simulink library "wcdma_lib"  (Simulink 6.0)
settings: Solver=ode45  SolverMode=SingleTasking  StartTime=0.0  StopTime=10.0  RelTol=1e-3
values from neighbouring files (symbols this model uses):
  allocationssc = [1 1 1 1 1 1 1 1 1 1 1 1 ... (960 elements, 64x15)]    [wcdma_allocationssc.mat]
  crcSize = str2num(Vals{idxCrcSize})    [wcdma_initmaskphlayer.m]    (also in wcdma_loadinitmuxandcoding.m = [16 12]; wcdma_loadinitphlayer.m = [16 12])
  errorCorr = (errorCorr>2)*2 + (errorCorr<3).*errorCorr    [wcdma_initmaskphlayer.m]    (also in wcdma_loadinitmuxandcoding.m = [2 2]; wcdma_loadinitphlayer.m = [2 2])
  i = [1:2:numSamp-1]'    [cdma2000_inttable.m]
  numBitsCodeWord = cond.*Zmin + not(cond).*numBitsCodeWord    [wcdma_concseg.m]    (also in wcdma_loadinitmuxandcoding.m = [260 122])
  numBitsFirstInt = numBitsRM + deltaNimax    [wcdma_initmaskphlayer.m]    (also in wcdma_loadinitmuxandcoding.m = [686 308])
  numBitsRF = numBitsFirstInt./(tti/10)    [wcdma_initmaskphlayer.m]    (also in wcdma_loadinitmuxandcoding.m = [343 77]; wcdma_loadinitphlayer.m = [343 77])
  numBitsTrCh = (trBlkSize+crcSize)*diag(numTrBlks)    [wcdma_concseg.m]    (also in wcdma_loadinitmuxandcoding.m = [260 112])
  numCodeWords = ceil(numBitsTrCh./Zmax(errorCorr+1))    [wcdma_concseg.m]    (also in wcdma_loadinitmuxandcoding.m = [1 1])
  numPadBits = (numBitsCodeWord.*numCodeWords)-numBitsTrCh    [wcdma_concseg.m]    (also in wcdma_loadinitmuxandcoding.m = [0 0])
  numPhCH = str2num(Vals{idxNumPhCH})    [wcdma_initmaskphlayer.m]    (also in wcdma_loadinitmuxandcoding.m = 1; wcdma_loadinitphlayer.m = 1)
  numTrBlks = trBlkSetSize./trBlkSize    [wcdma_concseg.m]    (also in wcdma_initmaskphlayer.m; wcdma_loadinitmuxandcoding.m = [1 1]; wcdma_loadinitphlayer.m = [1 1])
  overSampling = str2num(Vals{idxOverSampling})    [wcdma_initmaskphlayer.m]    (also in wcdma_initmaskspreadandmod.m; wcdma_loadinitphlayer.m = 8; wcdma_loadinitspreadandmod.m = 8)
  powerVector = str2num(Vals{idxPowerVector})    [wcdma_initmaskphlayer.m]    (also in wcdma_initmaskspreadandmod.m; wcdma_loadinitphlayer.m = [-5.5 -10 -15 -12 -12]; wcdma_loadinitspreadandmod.m = [-5.5 -10 -15 -12 -12])
  sprdFactor = wcdma_slotformattable(slotFormat+1,2)    [wcdma_checkparamstxant.m]    (also in wcdma_initmaskphlayer.m = slotformattable(slotFormat+1,2); wcdma_initmaskspreadandmod.m = slotformattable(slotFormat+1,2); wcdma_loadinitphlayer.m = 128; wcdma_loadinitspreadandmod.m = 128)
  tti = str2num(Vals{idxTti})    [wcdma_initmaskphlayer.m]    (also in wcdma_loadinitmuxandcoding.m = [20 40]; wcdma_loadinitphlayer.m = [20 40])
undefined symbols (not defined in the file or in its folder): hadamard, numSymbOut
libraries: wcdma_lib x122, dspsrcs4 x39, dspsigops x30, commseqgen2 x24, dspindex x20, dspbuff3 x19, dspmathops x16, simulink x10, dspsigattribs x7, commutil2 x6, dspmtrx3 x6, commblkintrlv2 x6
(part 1 of 3)
settings Model: Creator=arodrigu  LastModifiedBy=arodrigu  ProdHWDeviceType=Specified
settings DataIOCC: SignalLoggingName=logsOut
settings OptimizationCC: BooleanDataType=off
settings DebuggingCC: CheckExecutionContextPreStartOutputMsg=on  CheckExecutionContextRuntimeOutputMsg=on  SolverPrmCheckMsg=none
settings HardwareCC: ProdHWDeviceType=Specified  TargetUnknown=on
settings ModelReferenceCC: UpdateModelReferenceTargets=IfOutOfDate
settings GRTTargetCC: LifeSpan=inf
settings SFSimCC: SFSimApplyToAllLibs=on  SFSimBuildMode=Incremental

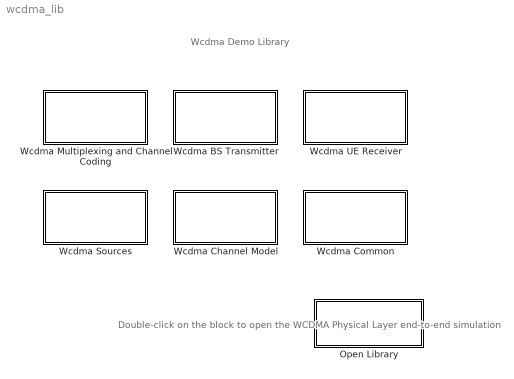
== system wcdma_lib ==
  note: Wcdma Demo Library
  note: Double-click on the block
      | to open the WCDMA Physical
      | Layer end-to-end simulation
  Open Library : Subsystem  EnableExecutionContextPropagation=on
      settings: OpenFcn=open('wcdma_phlayer.mdl');
      mask Display: disp('WCDMA PhLayer\nEnd-to-End\nSimulation')
  Wcdma BS Transmitter : Subsystem  EnableExecutionContextPropagation=on
      mask Type: Wcdma BS Tx
      mask Display: disp('Wcdma \nBS \nTransmitter');
  Wcdma Channel Model : Subsystem  EnableExecutionContextPropagation=on
      mask Type: Wcdma Common
      mask Display: disp('Wcdma \nChannel Model');
  Wcdma Common : Subsystem  EnableExecutionContextPropagation=on
      mask Type: Wcdma Common
      mask Display: disp('Wcdma \nCommon Blocks');
  Wcdma Multiplexing and Channel Coding : Subsystem  EnableExecutionContextPropagation=on
      mask Display: disp('Wcdma\nMultiplexing\nand Channel coding');
  Wcdma Sources : Subsystem  EnableExecutionContextPropagation=on
      mask Type: Wcdma Sources
      mask Display: disp('Wcdma \nSources');
  Wcdma UE Receiver : Subsystem  EnableExecutionContextPropagation=on
      mask Type: Wcdma UE Rx
      mask Display: disp('Wcdma \nUE \nReceiver');

== system wcdma_lib/Open Library ==
  note: This subsystem is intentionally left empty

== system wcdma_lib/Wcdma BS Transmitter ==
  note: Wcdma BS Transmitter
  Complex Spreading Multiplication : Subsystem  EnableExecutionContextPropagation=on  mask(Complex Spreading){sprdFactor=256}
      mask prompts: sprdFactor "Spreading Factor (SF):"
  Wcdma BS Tx Antenna : Subsystem  EnableExecutionContextPropagation=on  mask(Wcdma BS Tx Antenna){slotFormat=11, dpchCode=123, scrCode=[63 0], powerVector=[-8.8 -10 -15 -12 -12], numTapsRRC=96, overSampling=8, checkparams=off}
      mask prompts: slotFormat "Slot Format (0..16):"; dpchCode "DPCH Code number (0..Spreading Factor -1):"; scrCode "Scrambling Code [Scr Code Grup(0..63) Primary Code(0..7)]:"; powerVector "Power for [DPCH, P-CPICH, PICH, P-CCPCH, SCH] in dB:"; numTapsRRC "Number of Filter Taps for RRC filters:"; overSampling "Oversampling Factor:"; checkparams "Check here to validate parameters."
      mask help:
      | After combining the different transport channels into physical channels, data is sent to the Downlink Base Station Tranmitter Antenna in the form of slots.
      |
      | At the Transmitter antenna, data is first spread by a real-value orthogonal signature code for channel separation and then is scrambled by a complex-valued Gold Code Sequence.
      |
      | Finally other channels that are also transmitted during a connection are added together with different weights to create the waveform that is sent through the channel after applying the transmitter pulse shaping filter.
      |
      | For details on the implementation, see 3GPP TS 25.101, 3GPP TS 25.211 and 3GPP TS 25.213.
      mask init:
      | if slotFormat < 2
      | numChipsOut = 512;
      | else
      | numChipsOut = 256;
      | end
      | if(checkparams == 1)
      | wcdma_checkparamstxant.m;
      | end
      mask Help:
      | <p>After combining the different transport channels into physical channels, data is sent to the Downlink Base Station Tranmitter Antenna in the form of slots. </p>
      | 
      | <p>At the Transmitter antenna, data is first spread by a real-value orthogonal signature code for channel separation and then is scrambled by a complex-valued Gold Code Sequence.</p>
      | 
      | <p>Finally other channels that are also transmitted during a connection are added together with different weights to create the waveform that is sent through the channel after applying the transmitter pulse shaping filter. </p>
      | 
      | <p>For details on the implementation, see <a href="http://www.3gpp.org/specs/download.htm">3GPP TS.101 </a>, <a href="http://www.3gpp.org/specs/download.htm"> 3GPP TS 25.211</a> and <a href="http://www.3gpp.org/specs/download.htm"> 3GPP TS 25.213</a>.</p>
      mask Display: disp('Wcdma BS Tx\nAntenna');
  Wcdma DL Common  Channels Generator : Subsystem  EnableExecutionContextPropagation=on  mask(Wcdma DL Common Channels Generator){antenna=1, numSymbOut=1, st=1/15e3}
      mask prompts: antenna "Select Antenna (1-2):"; numSymbOut "Number of Symbols per Output:"; st "Symbol Time (Ts):"
      mask help: This block generates P-CPICH (Primary Common Pilot Generator), PICH (Paging Indicator Channel) and P-CCPCH (Primary-Common Control Physical Channel).
  Wcdma DPCH IQ Mapping : Subsystem  EnableExecutionContextPropagation=on
      mask Type: Wcdma DPCH Spreading
      mask Description: Each pair of DPCH bits is serial-to-parallel converted and mapped to an I and Q branch. Even numbered symbols are mapped to I branch whereas odd numbered are mapped to Q branch.
      mask Display: disp('DPCH IQ \nMapping')
  Wcdma Power Adjustment : Subsystem  EnableExecutionContextPropagation=on  mask(Wcdma Power Adjustment){powerVector=powerVector}
      mask prompts: powerVector "Power for [DPCH, P-CPICH, PICH, P-CCPCH, SCH] in dB:"
      mask help:
      | Using the power gains specified on the mask of the block, applies the corresponding weight to the different channels.
      |
      | The power settings for the OCNS are such that the total transmit power spectral density of the Node B adds to one, as is specified in Annex C of the 3GPP TS. 25.101 document.
      mask Display: disp('Wcdma\nPower\n Adjustment');
  Wcdma Power Settings : Subsystem  EnableExecutionContextPropagation=on  mask(Wcdma Power Settings){powerVector=powerVector}
      mask prompts: powerVector "Power for [DPCH, P-CPICH, PICH, P-CCPCH, SCH] in dB:"
  Wcdma SCH Multiplexer : Subsystem  EnableExecutionContextPropagation=on  mask(Wcdma SCH Multiplexer){numChipsOut=numSymbOut*256}
      mask prompts: numChipsOut "Number of Chips per Output:"
      mask help: Perform SCH multiplexing according to TS 25.211. The Primary CCPCH is not transmitted during the first 256 chips of each slot. Instead Primary and Secondary SCH are transmitted during this period..
      mask init:
      | numSymbOut = numChipsOut/256;
  Wcdma Scrambling : Subsystem  EnableExecutionContextPropagation=on  mask(Wcdma Scrambling){scrCode=[0 0], numChipsOut=256}
      mask prompts: scrCode "Scrambling Code [Scr Code Grup(0..63) Primary Code(0..7)]:"; numChipsOut "Number of Chips per Output:"
      mask help: Performs scrambling of the complex-valued input signal using a long Gold Code Sequence whose period is truncated to 10 ms. The same sequence is used by all the channels in the cell.
      mask Display: disp('Wcdma\nScrambling');
  Wcdma Spreading : Subsystem  EnableExecutionContextPropagation=on  mask(Wcdma Spreading){sprdFactor=256, dpchCode=256-1, codeVector=[0 4 1], numChipsOut=256}
      mask prompts: sprdFactor "DPCH Spreading Factor :"; dpchCode "DPCH Code number :"; codeVector "Common Channels Code Number Vector (P-CPICH, PICH, P-CCPCH)"; numChipsOut "Number of Chips per Output:"
      mask help:
      | Performs spreading (also referred as channelization) of the complex-valuee input sequence by a real-valued orthogonal sequence whose indices are set on the mask of the block.
      |
      | This operation transform every symbol of data into a given number of chips. The number of chips per symbol is called Spreading Factor.
      |
      | The orthogonal codes specified by 3GPP TS 25.213 are Orthogonal Variable Spreading Factor (OVSF) codes.
      mask Display: disp('Wcdma\nSpreading')

== system wcdma_lib/Wcdma Channel Model ==
  note: Wcdma Channel Models
  AWGN : Subsystem  EnableExecutionContextPropagation=on
      mask Display: disp('Wcdma Channel Model:\nAWGN Channel');
  Multipath+AWGN : Subsystem  EnableExecutionContextPropagation=on
      mask Display: disp('Wcdma Channel Model:\nMultipath-AWGN Channel');
  No Channel : Subsystem  EnableExecutionContextPropagation=on
      mask Display: disp('Wcdma Channel Model:\nNo Channel');
  Wcdma Channel Models : Subsystem  BlockChoice=AWGN  EnableExecutionContextPropagation=on
      settings: TemplateBlock=self  MemberBlocks=AWGN,Multipath+AWGN,No Channel

== system wcdma_lib/Wcdma Common ==
  note: Wcdma Common Blocks
  BLER Calculation : Subsystem  EnableExecutionContextPropagation=on  mask(BLER Calculation){trBlkSetSize=[244 100], tti=[20 40], numBitsDelay=[488 200]}
      mask prompts: trBlkSetSize "Transport Block Set Size:"; tti "TTI (in ms):"; numBitsDelay "Number of Bits Delay:"
      mask init:
      | numTrBlksDelay = numBitsDelay./trBlkSetSize;
      | [m,i] = min(numTrBlksDelay.* tti);
      | minNumTrBlksDelay = numTrBlksDelay(i);
      | [m,i] = min(tti);
      mask Display: disp('BLER\nCalculation');
  "Complex Unipolar to Bipolar " : Subsystem  EnableExecutionContextPropagation=on  mask(Unipolar to Bipolar Converter){M=2, polarity=Negative}
      mask prompts: M "M-ary number:"
      mask help: Convert a unipolar signal in the range [0, M-1], where M is the M-ary number, into a bipolar signal.
      mask init:
      | if strcmp(polarity, 'Negative')
      |    pole = -1;
      | else
      |    pole = 1;
      | end
      mask Help: helpview(commbhelp);
      mask StyleString: edit,popup(Positive|Negative)
      mask Display: disp(' Complex \nUnipolar to \nBipolar');
  Complex  Bipolar to Unipolar : Subsystem  EnableExecutionContextPropagation=on  mask(Bipolar to Unipolar Converter){M=2, polarity=Negative}
      mask prompts: M "M-ary number:"
      mask help: Convert a bipolar signal into a unipolar signal in the range [0, M-1], where M is the M-ary number.
      mask init:
      | if strcmp(polarity, 'Negative')
      |    pole = -1;
      | else
      |    pole = 1;
      | end
      mask Help: helpview(commbhelp);
      mask StyleString: edit,popup(Positive|Negative)
      mask Display: disp('Bipolar to\nUnipolar\nConverter');
  Energy Measurement : Subsystem  EnableExecutionContextPropagation=on
      mask Display: disp('Energy')
  Hadamard Matrix : Subsystem  EnableExecutionContextPropagation=on  mask(Hadamard Matrix){order=8}
      mask Display: disp('256-Hadamard\nMatrix');
  Low Pass Filter : Subsystem  EnableExecutionContextPropagation=on  mask(Channel Estimation low pass filter){N=2, Wn=1/4, outputBufInitCond=0}
      mask prompts: N "Order of the Filter:"; Wn "Cut-off Frequency"; outputBufInitCond "Output buffer initial conditions:"
      mask help: KAISER window Low Pass filter
      mask init:
      | h=fir1(N,Wn,kaiser(N+1,4))';
      mask Display: plot( 1:prod( size( h)), h);
  Normalize Ec : Subsystem  EnableExecutionContextPropagation=on
      mask Description: This block normalizes the energy per sample of the input sequence.
      mask Display: disp('Normalize\nEc');
  dB-Linear Conversion : Subsystem  EnableExecutionContextPropagation=on
      mask Type: dB Conversion
      mask Description: Convert dB to Linear
      mask Display: disp('dB to linear')

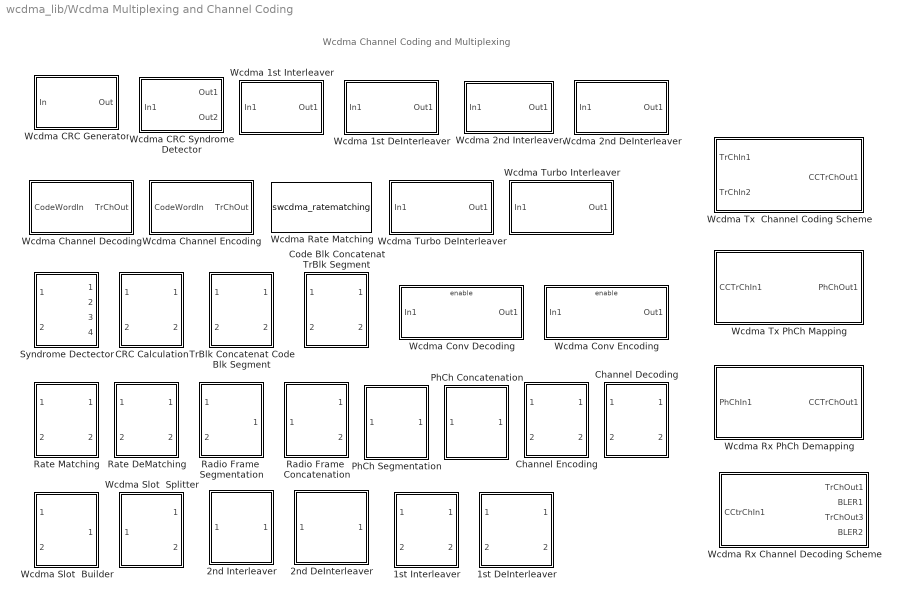
== system wcdma_lib/Wcdma Multiplexing and Channel Coding ==
  note: Wcdma Channel Coding and Multiplexing
  1st DeInterleaver : Subsystem  EnableExecutionContextPropagation=on
      mask Type: Wcdma 1st Interleaver
      mask Display: disp('1st\nDeInterleaver');
  1st Interleaver : Subsystem  EnableExecutionContextPropagation=on
      mask Type: Wcdma 1st Interleaver
      mask Display: disp('1st\nInterleaver');
  2nd DeInterleaver : Subsystem  EnableExecutionContextPropagation=on
      mask Type: 2nd DeInterleaver
      mask Display: disp('2nd\nDeinterleaver');
  2nd Interleaver : Subsystem  EnableExecutionContextPropagation=on
      mask Type: 2nd Interleaver
      mask Display: disp('2nd\nInterleaver');
  CRC Calculation : Subsystem  EnableExecutionContextPropagation=on
      mask Type: CRC Calculation
      mask Display: disp('Wcdma\nCRC\nCalculation');
  Channel Decoding : Subsystem  EnableExecutionContextPropagation=on
      mask Type: Channel Decoding
      mask Display: disp('Channel\nDecoding');
  Channel Encoding : Subsystem  EnableExecutionContextPropagation=on
      mask Type: Channel Encoding
      mask Display: disp('Channel\nEncoding');
  Code Blk Concatenat TrBlk Segment : Subsystem  EnableExecutionContextPropagation=on  mask(Code BlK Concatenation and TrBlk Segmentation){trBlkSetSize=[488 200], trBlkSize=[244 100], crcSize=[16 12]}
      mask prompts: trBlkSetSize "Transport Block Set Size:"; trBlkSize "Transport Block Size:"; crcSize "Size of CRC Vector {24, 16, 12, 8, 0}:"
      mask help:
      | The function :
      |
      | [numBitsTrCh, numPadBits, numCodeWords, numBitsCodeWord] = wcdma_concseg(trBlkSetSize,trBlkSize,crcSize, errorCorr);
      |
      | computes the number of bits per Transport Channel, number of Padding Bits, number of Code Words as well as the number bits in each Code Word.
      mask init:
      | numTrBlks = trBlkSetSize./trBlkSize;
      mask Display: disp('Code Blk\nConcatenat\nTrBlk\nSegment');
  PhCh Concatenation : Subsystem  EnableExecutionContextPropagation=on
      mask Type: PhCh Concatenation
      mask Display: disp('PhCh\nConcat');
  PhCh Segmentation : Subsystem  EnableExecutionContextPropagation=on
      mask Type: PhCh Segmentation
      mask Display: disp('PhCh\nSegment');
  Radio Frame  Concatenation : Subsystem  EnableExecutionContextPropagation=on  mask(Radio Frame Concatenation){numBits=[260 112], tti=[20 40], checkDelay=off}
      mask prompts: numBits "Number of Bits per Transport Channel:"; tti "TTI (in ms):"; checkDelay "Check here if Rx Antenna is connected in the model."
      mask init:
      | numBitsRF = numBits./(tti/10);
      mask Display: disp('Radio\nFrame\nConcat');
  Radio Frame  Segmentation : Subsystem  EnableExecutionContextPropagation=on
      mask Type: Radio Frame Segmentation
      mask Display: disp('Radio\nFrame\nSegment');
  Rate DeMatching : Subsystem  EnableExecutionContextPropagation=on
      mask Type: Rate DeMatching
      mask Display: disp('Rate\nDematching');
  Rate Matching : Subsystem  EnableExecutionContextPropagation=on
      mask Type: Rate Matching
      mask Display: disp('Rate\nMatching');
  Syndrome Dectector : Subsystem  EnableExecutionContextPropagation=on
      mask Type: Syndrome Detector
      mask Display: disp('Wcdma\nSyndrome\nDetector');
  TrBlk Concatenat Code Blk Segment : Subsystem  EnableExecutionContextPropagation=on  mask(TrBlk Concatenation and Code Blk Segmentation){numBitsTrCh=[488 200], numPadBits=[0 0], numBitsCodeWord=[0 0]}
      mask prompts: numBitsTrCh "Number of Bits per Transport Channel:"; numPadBits "Number of Padding Bits:"; numBitsCodeWord "Number of Bits per Code Word:"
      mask help:
      | The function :
      |
      | [numBitsTrCh, numPadBits, numCodeWords, numBitsCodeWord] = wcdma_concseg(trBlkSetSize,trBlkSize,crcSize, errorCorr);
      |
      | computes the number of bits per Transport Channel, number of Padding Bits, number of Code Words as well as the number bits in each Code Word.
      mask Display: disp('TrBlk\nConcatenat\nCode Blk\n Segment');
  Wcdma 1st DeInterleaver : Subsystem  EnableExecutionContextPropagation=on  mask(Wcdma 1st Deinterleaver){numBits=244, tti=20}
      mask prompts: numBits "Number of Input Bits:"; tti "TTI (in ms):"
      mask help: Interleave the input vector by writing the elements into a matrix row-by-row, performing inter-column permutation by using an specific pattern defined in 3GPP TS 25.212 and reading them out column-by-column.
      mask init:
      | int_table = wcdma_firstinterleaver(numBits, tti);
      mask Display: disp('Wcdma\n1st Deinterleaver')
  Wcdma 1st Interleaver : Subsystem  EnableExecutionContextPropagation=on  mask(Wcdma 1st Interleaver){numBits=244, tti=20}
      mask prompts: numBits "Number of Input Bits:"; tti "TTI (in ms):"
      mask help: Interleave the input vector by writing the elements into a matrix row-by-row, performing inter-column permutation by using an specific pattern defined in 3GPP TS 25.212 and reading them out column-by-column.
      mask init:
      | int_table = wcdma_firstinterleaver(numBits, tti);
      mask Display: disp('Wcdma\n1st Interleaver')
  Wcdma 2nd DeInterleaver : Subsystem  EnableExecutionContextPropagation=on  mask(Wcdma 2nd DeInterleaver){numBits=520}
      mask prompts: numBits "Number of Input Bits:"
      mask help: Interleave the input vector by writing the elements into a matrix row-by-row, performing inter-column permutation by using an specific pattern defined in 3GPP TS 25.212 and reading them out column-by-column.
      mask init:
      | int_table = wcdma_secondinterleaver(numBits);
      mask Display: disp('Wcdma\n2nd DeInterleaver')
  Wcdma 2nd Interleaver : Subsystem  EnableExecutionContextPropagation=on  mask(Wcdma 2nd Interleaver){numBits=520}
      mask prompts: numBits "Number of Input Bits:"
      mask help: Interleave the input vector by writing the elements into a matrix row-by-row, performing inter-column permutation by using an specific pattern defined in 3GPP TS 25.212 and reading them out column-by-column.
      mask init:
      | int_table = wcdma_secondinterleaver(numBits);
      mask Display: disp('Wcdma\n2nd Interleaver')
  Wcdma Channel Decoding : Subsystem  EnableExecutionContextPropagation=on  mask(Wcdma Channel Decoding){errorCorr=2, numBitsCodeWord=488, numCodeWords=1, tti=20}
      mask prompts: errorCorr "Type of Error Protection {None=0, Conv 1/2=1, Conv 1/3=2, Turbo=3}:"; numBitsCodeWord "Number of Bits per Code Word:"; numCodeWords "Number of Code Words:"; tti "TTI (in ms):"
      mask init:
      | switch(errorCorr)
      | case 0 % No Channel Coding
      |     codeRate = 1;
      |     tailBits = 0;
      |     selectBits = [1:numBitsCodeWord*numCodeWords];
      |     enableEnc = 0;
      | case 1 % Conv Coding 1/2
      |     codeRate = 2;
      |     tailBits = 8;
      |     selectBits = (numBitsCodeWord+tailBits)*codeRate*numCodeWords+[1:numBitsCodeWord];
      |     enableEnc = 1;
      | case 2 % Conv Coding 1/3
      |     codeRate = 3;
      |     tailBits = 8;
      |     selectBits = (numBitsCodeWord+tailBits)*codeRate*numCodeWords+[1:numBitsCodeWord];
      |     enableEnc = 1;
      | case 3 % Turbo Coding
      |     enableEnc = 0;
      |      % Not currently implemented
      | end
      mask Display: disp('Wcdma\nChannel Decoding');
  Wcdma Channel Encoding : Subsystem  EnableExecutionContextPropagation=on  mask(Wcdma Channel Encoding){errorCorr=2, numBitsCodeWord=488, numCodeWords=1, tti=20}
      mask prompts: errorCorr "Type of Error Protection {None=0, Conv 1/2=1, Conv 1/3=2, Turbo=3}:"; numBitsCodeWord "Number of Bits per Code Word:"; numCodeWords "Number of Code Words:"; tti "TTI (in ms):"
      mask help: Performs Channel encoding to each transport channel separately.
      mask init:
      | switch(errorCorr)
      | case 0 % No Channel Coding
      |     codeRate = 1;
      |     tailBits = 0;
      |     selectBits = [1:numBitsCodeWord];
      |     enableEnc = 0;
      | case 1 % Conv Coding 1/2
      |     codeRate = 2;
      |     tailBits = 8;
      |     selectBits = numBitsCodeWord+[1:(numBitsCodeWord+tailBits)*codeRate*numCodeWords];
      |     enableEnc = 1;
      | case 2 % Conv Coding 1/3
      |     codeRate = 3;
      |     tailBits = 8;
      |     selectBits = numBitsCodeWord+[1:(numBitsCodeWord+tailBits)*codeRate*numCodeWords];
      |     enableEnc = 1;
      | case 3 % Turbo Coding
      |     enableEnc = 0;
      |      % Not currently implemented
      | end
      mask Help: Performs Channel encoding to each transport channel separately.
      mask Display: disp('Wcdma\nChannel Encoding');
  Wcdma Rate Matching : S-Function  FunctionName=swcdma_ratematching  Parameters=deltaNimax, numBits, errorCorr, checkRM  mask(Wcdma Rate Matching){idxTrCh=1, numBits=[804 360], RMAttribute=[256 256], tti=[20 40], errorCorr=[2 2], posTrCh=0, slotFormat=11, numPhCH=1, checkRM=off}
      mask prompts: idxTrCh "Index of the current Transport Channel {1..8}:"; numBits "Number of Bits per Transport Channel:"; RMAttribute "Rate Matching Attribute:"; tti "TTI (in ms):"; errorCorr "Type of Error Protection {None=0, Conv 1/2=1, Conv 1/3=2, Turbo=3}:"; posTrCh "Position of TrCH in Radio Frame {Fixed=0, Flexible=1}:"; slotFormat "Slot Format (0..16):"; numPhCH "Number of Physical Channels"; checkRM "Check for Rate Dematching"
      mask init:
      | deltaNimax = wcdma_ratematchinginit(numBits, tti, RMAttribute, posTrCh, slotFormat, numPhCH);
      | 
      | deltaNimax = deltaNimax(idxTrCh);
      | numBits = numBits(idxTrCh);
      | errorCorr = errorCorr(idxTrCh);
      mask StyleString: popup(1|2|3|4|5|6|7|8),edit,edit,edit,edit,edit,edit,edit,checkbox
      mask Display: disp('Wcdma\nRate Matching');
  Wcdma Turbo DeInterleaver : Subsystem  EnableExecutionContextPropagation=on  mask(Wcdma Turbo DeInterleaver){numBitsCodeWord=244}
      mask prompts: numBitsCodeWord "Number of Bits per Code Word:"
      mask help: Interleave the input vector by writing the elements into a matrix row-by-row, performing inter-column permutation by using an specific pattern defined in 3GPP TS 25.212 and reading them out column-by-column.
      mask init:
      | int_table = wcdma_turbointerleaver(numBitsCodeWord);
      mask Display: disp('Wcdma\nTurbo DeInterleaver')
  Wcdma Turbo Interleaver : Subsystem  EnableExecutionContextPropagation=on  mask(Wcdma Turbo Interleaver){numBitsCodeWord=244}
      mask prompts: numBitsCodeWord "Number of Bits per Code Word:"
      mask help: Interleave the input vector by writing the elements into a matrix row-by-row, performing inter-column permutation by using an specific pattern defined in 3GPP TS 25.212 and reading them out column-by-column.
      mask init:
      | int_table = wcdma_turbointerleaver(numBitsCodeWord);
      mask Display: disp('Wcdma\nTurbo Interleaver')
  Wcdma CRC Generator : Subsystem  EnableExecutionContextPropagation=on  mask(Wcdma CRC Generator){bits=24, iniStates=0, dataFrames=100}
      mask prompts: bits "CRC Size {24, 16, 12, 8, 0}:"; iniStates "Initial States:"; dataFrames "Number of Checks per Frame:"
      mask help:
      | Generate the CRC bits according to the generator polynomials specified in 3G TS 25.212 and append them to the input data frames.
      |
      | The input must be a frame-based column vector and can comprise of multiple data frames as specified by the input data frames parameter.
      mask init:
      | if bits == 24
      |    genPoly = [1 1 0 0 0 0 0 0 0 0 0 0 0 0 0 0 0 0 1 1 0 0 0 1 1];
      | elseif bits==16
      |    genPoly = [1 0 0 0 1 0 0 0 0 0 0 1 0 0 0 0 1];
      | elseif bits==12
      |    genPoly = [1 1 0 0 0 0 0 0 0 1 1 1 1];
      | elseif bits==8
      |    genPoly = [1 1 0 0 1 1 0 1 1];
      | else
      |    genPoly = [1];
      | end
      mask Display: disp('Wcdma CRC\nGenerator');
  Wcdma CRC Syndrome Detector : Subsystem  EnableExecutionContextPropagation=on  mask(Wcdma CRC Syndrome Detector){bits=24, iniStates=0, dataFrames=100}
      mask prompts: bits "No of Bits:"; iniStates "Initial states:"; dataFrames "Output Data Frames:"
      mask help:
      | Wcdma CRC syndrome detector removes the redundant bits from the input data frames as per the generator polynomials specified in 3G TS 25.212 and checks the input data for any frame errors.
      |
      | The input must be a frame-based column vector and can comprise of multiple data frames as specified by the output data frames parameter.
      mask init: same as wcdma_lib/Wcdma Multiplexing and Channel Coding/Wcdma CRC Generator
      mask Display: disp('Wcdma CRC\nSyndrome\nDetector');
  Wcdma Conv Decoding : Subsystem  TreatAsAtomicUnit=on  EnableExecutionContextPropagation=on  mask(Wcdma Convolutional Decoding){errorCorr=2, numBitsCodeWord=488, numCodeWords=1}
      mask prompts: errorCorr "Type of Error Protection {None=0, Conv 1/2=1, Conv 1/3=2, Turbo=3}:"; numBitsCodeWord "Number of Bits per Code Word:"; numCodeWords "Number of Code Words:"
      mask init:
      | % Default Case
      | codeRate = 1;
      | tailBits = 0;
      | trellis = poly2trellis(9, [561 753]);
      | if errorCorr == 1 % Conv Coding 1/2
      |     codeRate = 2;
      |     tailBits = 8;
      |     trellis = poly2trellis(9, [561 753]);
      | elseif errorCorr == 2 % Conv Coding 1/3
      |     codeRate = 3;
      |     tailBits = 8;
      |     trellis = poly2trellis(9, [557 663 711]);
      | end
      mask Display: disp('Wcdma\n Convolutional Decoding');
  Wcdma Conv Encoding : Subsystem  TreatAsAtomicUnit=on  EnableExecutionContextPropagation=on  mask(Conv Encoding){errorCorr=2, numBitsCodeWord=488, numCodeWords=1}
      mask prompts: errorCorr "Type of Error Protection {None=0, Conv 1/2=1, Conv 1/3=2, Turbo=3}:"; numBitsCodeWord "Number of Bits per Code Word:"; numCodeWords "Number of Code Words:"
      mask init:
      | % Default Case
      | codeRate = 2;
      | tailBits = 8;
      | trellis = poly2trellis(9, [561 753]);
      | 
      | if errorCorr == 2 % Conv Coding 1/3
      |     codeRate = 3;
      |     trellis = poly2trellis(9, [557 663 711]);
      | end
      mask Display: disp('Wcdma\nConvolutional Encoding');
  Wcdma Rx Channel Decoding Scheme : Subsystem  EnableExecutionContextPropagation=on  mask(Wcdma DL Rx Channel Decoding Scheme){trBlkSetSize=[244 100], trBlkSize=[244 100], tti=[20 40], crcSize=[16 12], errorCorr=[2 2], RMAttribute=[256 256], posTrCh=0, numPhCH=1, slotFormat=11, checkParams=on}
      mask prompts: trBlkSetSize "Transport Block Set Size:"; trBlkSize "Transport Block Size:"; tti "TTI (in ms) {10, 20, 40, 80):"; crcSize "CRC Size {24, 16, 12, 8, 0}:"; errorCorr "Type of Error Protection {None=0, Conv 1/2=1, Conv 1/3=2, Turbo=3}:"; RMAttribute "Rate Matching Attribute:"; posTrCh "Position of TrCH in Radio Frame {Fixed=0, Flexible=1}:"; numPhCH "Number of PhCH:"; slotFormat "Slot Format (0..16):"; checkParams "Check here to validate parameters."
      mask help: As specified in the 3GPP TS.212 V3.6.0 document, the Downlink channel decoding scheme consists of error detection, error correction, rate matching, interleaving and transport channels splitting from the Coded Composite Transport Channel (CCTrCh).
      mask init:
      | numTrBlks = trBlkSetSize./trBlkSize;
      | [numBitsTrCh, numPadBits, numCodeWords, numBitsCodeWord] = wcdma_concseg(trBlkSetSize,trBlkSize,crcSize, errorCorr);
      | codeRate = errorCorr+1 - (errorCorr == 3);
      | tailBits = 8 *(errorCorr ~=0);
      | numBitsRM = codeRate.*(numBitsCodeWord+tailBits).*numCodeWords;
      | 
      | deltaNimax = wcdma_ratematchinginit(numBitsRM, tti, RMAttribute, posTrCh, slotFormat, numPhCH);
      | numBitsFirstInt = numBitsRM + deltaNimax;
      | numBitsRF = numBitsFirstInt./(tti/10);
      | 
      | if(checkParams == 1)
      | wcdma_checkparamserrorcorr;
      | end
      mask Help: As specified in the <a href="http://www.3gpp.org/specs/download.htm">3GPP TS.212 V3.6.0</a>  document, the <b> Downlink channel decoding scheme </b> consists of error detection, error correction, rate matching, interleaving and transport channels splitting from the <i>Coded Composite Transport Channel (CCTrCh)</i>.
      mask Display: disp('Wcdma DL Rx\nChannel Decoding Scheme');
  Wcdma Rx PhCh Demapping : Subsystem  EnableExecutionContextPropagation=on  mask(Wcdma Rx Physical Channel Demapping){numBitsRF=[420 80], numPhCH=1, slotFormat=11, checkParams=on}
      mask prompts: numBitsRF "Number of Bits per CCTrCh:"; numPhCH "Number of PhCH:"; slotFormat "Slot Format (0..16):"; checkParams "Check here to validate parameters."
      mask help: As described in the 3GPP TS25.212 V3.6.0 document, the Downlink physical channel demapping is in charge of splitting and organizing the bits of the demodulated physical channel in order to reconstruct the Coded Composite Transport Channel (CCTrCh).
      mask init:
      | if(checkParams == 1) wcdma_checkparamsphmap;
      | end
      mask Help: As described in the <a href="http://www.3gpp.org/specs/download.htm">3GPP TS.212 V3.6.0</a>  document, the <b>Downlink physical channel demapping</b> is in charge of splitting and organizing the bits of the demodulated physical channel in order to reconstruct the <i>Coded Composite Transport Channel (CCTrCh).</i>
      mask Display: disp('Wcdma Rx\n Physical Channel Demapping');
  Wcdma Slot  Builder : Subsystem  EnableExecutionContextPropagation=on  mask(Wcdma Slot Builder){slotFormat=11}
      mask prompts: slotFormat "Slot Format (0..16):"
      mask init:
      | % Load Slot format table
      | load wcdma_slotformattable;
      | 
      | % Get variables
      | Ndata1 = slotformattable(slotFormat+1,4);
      | Ndata1prima = Ndata1 + (Ndata1 == 0);
      | Ndata2 = slotformattable(slotFormat+1,5);
      | Ntpc = slotformattable(slotFormat+1,6);
      | Ntfci = slotformattable(slotFormat+1,7);
      | Ntfciprima = Ntfci + (Ntfci == 0);
      | Npilot = slotformattable(slotFormat+1,8);
      | 
      | % Puncturing Pattern
      | punctPattern = [(Ndata1~=0)*ones(1,Ndata1prima) ones(1,Ntpc) (Ntfci~=0)*ones(1,Ntfciprima) ones(1,Ndata2) ones(1,Npilot)]';
      mask Display: disp('Wcdma\nSlot Builder');
  Wcdma Slot  Splitter : Subsystem  EnableExecutionContextPropagation=on  mask(Wcdma Slot Splitter){slotFormat=11, numSlotDelay=3}
      mask prompts: slotFormat "Slot Format (0..16):"; numSlotDelay "Number of Slots Delay after demodulation:"
      mask init:
      | % Load Slot format table
      | load wcdma_slotformattable;
      | 
      | % Get variables
      | Ndata1 = slotformattable(slotFormat+1,4);
      | Ndata1prima = Ndata1 + (Ndata1 == 0);
      | Ndata2 = slotformattable(slotFormat+1,5);
      | Ntpc = slotformattable(slotFormat+1,6);
      | Ntfci = slotformattable(slotFormat+1,7);
      | Ntfciprima = Ntfci + (Ntfci == 0);
      | Npilot = slotformattable(slotFormat+1,8);
      | 
      | % Input to selector block
      | selectPattern = {[1:Ndata1prima],[Ndata1+1:Ndata1+Ntpc],...
      |         [Ndata1+Ntpc+1:Ndata1+Ntpc+Ntfciprima],...
      |         [Ndata1+Ntpc+Ntfci+1:Ndata1+Ntpc+Ntfci+Ndata2],...
      |         [Ndata1+Ntpc+Ntfci+Ndata2+1:Ndata1+Ntpc+Ntfci+Ndata2+Npilot]};
      | 
      | % Second Selector
      | selectPattern2 = {[1:Ndata1+Ndata2]+(Ndata1==0)};
      | 
      | % Compute Samples Delay introduced by demodulator
      | samplesDelay = (Ndata1+Ndata2)*numSlotDelay;
      mask Display: disp('Wcdma\nSlot Splitter');
  Wcdma Tx PhCh Mapping : Subsystem  EnableExecutionContextPropagation=on  mask(Wcdma Tx Physical Channel Mapping){numBitsRF=[420 80], numPhCH=1, slotFormat=11, checkParams=on}
      mask prompts: numBitsRF "Number of Bits per CCTrCh:"; numPhCH "Number of PhCH:"; slotFormat "Slot Format (0..16):"; checkParams "Check here to validate parameters."
      mask help:
      | As described in the 3GPP TS25.212 V3.6.0 document, the Downlink physical channel mapping is in charge of organizing and multiplexing the bits of the Coded Composite Transport Channel (CCTrCh), which is the result of the concatenation of the different transport channels, into a Dedicated Physical Channel (DPCH) in the form of slots.
      |
      | Each slot of the Dedicated physical channel contains information data as well as control bits generated in by physical layer.
      mask init:
      | if(checkParams == 1)wcdma_checkparamsph;
      | end
      mask Help:
      | <p>As described in the <a href="http://www.3gpp.org/specs/download.htm">3GPP TS.212 V3.6.0</a>  document, the <b>Downlink physical channel mapping</b> is in charge of organizing and multiplexing the bits of the <i>Coded Composite Transport Channel (CCTrCh)</i>, which is the result of the concatenation of the different transport channels, into a <i>Dedicated Physical Channel (DPCH)</i> in the form of <i>slots </i>.</p>
      | 
      | <p>Each slot of the Dedicated physical channel contains information data as well as control bits generated in by physical layer.</p>
      mask Display: disp('Wcdma Tx\nPhysical Channel Mapping');
  Wcdma Tx  Channel Coding Scheme : Subsystem  EnableExecutionContextPropagation=on  mask(Wcdma DL Tx Channel Coding Scheme){trBlkSetSize=[244 100], trBlkSize=[244 100], tti=[20 40], crcSize=[16 12], errorCorr=[2 2], RMAttribute=[256 256], posTrCh=0, numPhCH=1, slotFormat=11, checkParams=on}
      mask prompts: trBlkSetSize "Transport Block Set Size:"; trBlkSize "Transport Block Size:"; tti "TTI (in ms) {10, 20, 40, 80):"; crcSize "CRC Size {24, 16, 12, 8, 0}:"; errorCorr "Type of Error Protection {None=0, Conv 1/2=1, Conv 1/3=2, Turbo=3}:"; RMAttribute "Rate Matching Attribute:"; posTrCh "Position of TrCH in Radio Frame {Fixed=0, Flexible=1}:"; numPhCH "Number of PhCH:"; slotFormat "Slot Format (0..16):"; checkParams "Check here to validate parameters."
      mask help: As specified in the 3GPP TS.212 V3.6.0 document, the Downlink channel encoding scheme consists of error detection, error correction, rate matching, interleaving and transport channels mapping onto the Coded Composite Transport Channel (CCTrCh).
      mask init: same as wcdma_lib/Wcdma Multiplexing and Channel Coding/Wcdma Rx Channel Decoding Scheme
      mask Help: As specified in the <a href="http://www.3gpp.org/specs/download.htm">3GPP TS.212 V3.6.0</a> document, the <b>Downlink channel encoding scheme </b> consists of error detection, error correction, rate matching, interleaving and transport channels mapping onto the <i>Coded Composite Transport Channel (CCTrCh)</i>.
      mask Display: disp('Wcdma DL Tx\nChannel Coding Scheme')

== system wcdma_lib/Wcdma Sources ==
  note: Wcdma Sources
  Channel Generator : Subsystem  EnableExecutionContextPropagation=on  mask(Channel Generator){rndSeed=12345, initDelay=0, numSymbOut=1, st=1/15e3}
      mask prompts: rndSeed "Random Seed:"; initDelay "Initial Delay (Units of Symbols):"; numSymbOut "Number of Symbols per Output:"; st "Symbol Time (Ts):"
  P-CPICH Generator : Subsystem  EnableExecutionContextPropagation=on  mask(Wcdma P-CPICH Generator){antenna=1, numSymbOut=1, st=1/15e3}
      mask prompts: antenna "Select Antenna:"; numSymbOut "Number of Symbols per Output:"; st "Symbol Time (Ts):"
      mask init:
      | %wcdma_pcpichgen(antenna, st);
      mask Display: disp('Wcdma P-CPICH\n Generator')
  Wcdma OCNS Generator : Subsystem  EnableExecutionContextPropagation=on  mask(Wcdma OCNS Generator){sprdFactor=256, numSymbOut=1, st=1/15e3}
      mask prompts: sprdFactor "OCNS Spreading Factor (SF):"; numSymbOut "Number of Symbols per Output:"; st "Symbol Time (Ts):"
      mask help: Generates ONCS interference as a combination of 16 dedicated data channels whose channelization codes, level settings and data timing offsets are specified by 3GPP standard (3GPP Ts 25.101).
      mask Display: disp('Wcdma OCNS\n Generator');
  Wcdma PSC Generator : Subsystem  EnableExecutionContextPropagation=on  mask(Wcdma PSC Generator){a_sch=-1}
      mask prompts: a_sch "Value of a {-1,1}:"
      mask Display: disp(' Primary SCH\nGenerator');
  Wcdma Pilot Bits Generator : Subsystem  EnableExecutionContextPropagation=on  mask(Wcdma Pilot Bits Generator){numPilotBits=6, frameSampTime=0.01}
      mask prompts: numPilotBits "Number of Pilot bits per slot:"; frameSampTime "Frame Sample Time:"
      mask init:
      | pilotBits = wcdma_pilotbitgenerator(numPilotBits);
      mask Display: disp('Wcdma\n Pilot Bits\nGenerator');
  Wcdma SCH  Generator : Subsystem  EnableExecutionContextPropagation=on  mask(Wcdma SCH Generator){scrGroup=0, a_sch=1}
      mask prompts: scrGroup "Scrambling Code Group (0..64):"; a_sch "Value of "a" {-1,1}:"
      mask help: Generate Synchronisation channel (SCH) as specified by 3GPP TS.25.213. The SCH is the results of combining two different subchannels: Primary SCH and Secondary SCH.
      mask Display: disp('Wcdma SCH\n Generator');
  Wcdma SSC Generator : Subsystem  EnableExecutionContextPropagation=on  mask(Wcdma SSC Generator){scrGroup=0, a_sch=-1}
      mask prompts: scrGroup "Scrambling Code Group (0..64):"; a_sch "Value of a {-1,1}:"
      mask init:
      | load wcdma_allocationssc.mat
      mask Display: disp(' Secondary SCH\nGenerator');
  Wcdma Scrambling Code Generator : Subsystem  EnableExecutionContextPropagation=on  mask(Wcdma Scr Code Generator){scrCode=[0 0], chipRate=3.84e6, numChipsOut=256}
      mask prompts: scrCode "Scrambling Code [Scr Code Grup(0..63) Primary Code(0..7)]:"; chipRate "Chip Rate (in s):"; numChipsOut "Number of Chips per Output:"
      mask Display: disp('Wcdma\nScr Code\nGenerator');

== system wcdma_lib/Wcdma UE Receiver ==
  note: Wcdma UE Receiver
  I&Q Demapping : Subsystem  EnableExecutionContextPropagation=on
      mask Type: I&Q Demapping
      mask Description: Transform complex signal into two serially concatenated real signals.
      mask Display: disp('DPCH IQ\nDemapping');
  Slot Rebuilder : Subsystem  EnableExecutionContextPropagation=on  mask(Wcdma Slot Rebuilder){numBits=40, totalDelay=44}
      mask prompts: numBits "Number of Bits per Slot:"; totalDelay "Total Receiver Delay"
      mask help:
      | Stores input symbols to generate slots of data.
      |
      | This block introduces an initial delay corresponding to one slot of data if the initial delay specified on the mask of the block is greater than 0,
      mask Display: disp('Slot\nRebuilder');
  Wcdma Channel Estimation : Subsystem  EnableExecutionContextPropagation=on  mask(Wcdma Channel Estimation){numTapsChEst=3, numChipsOut=256}
      mask prompts: numTapsChEst "Number of Filter Taps for Channel Estimation:"; numChipsOut "Number of Chips per Output:"
      mask help: Perform Channel Estimation
  Wcdma Correlator : Subsystem  TreatAsAtomicUnit=on  EnableExecutionContextPropagation=on  mask(Wcdma Correlator){sprdFactor=256}
      mask prompts: sprdFactor "Spreading Factor (SF):"
  Wcdma Data Derotation : Subsystem  EnableExecutionContextPropagation=on
      mask Type: Wcdma Data Derotation
      mask Description: Performs Data Derotation.
  Wcdma Orthogonal  Codes Generator : Subsystem  EnableExecutionContextPropagation=on  mask(Wcdma Orthogonal Codes Generator){sprdFactor=256, codeNumber=255, scrCode=[63 0], numChipsOut=256, st=1/15e3}
      mask prompts: sprdFactor "DPCH Spreading Factor (SF) :"; codeNumber "Code Number (k) :"; scrCode "Scrambling Code [Scr Code Grup(0..63) k(0..7)]:"; numChipsOut "Number of Chips per Output:"; st "Sampling Time:"
  Wcdma Rake Combiner : Subsystem  TreatAsAtomicUnit=on  EnableExecutionContextPropagation=on
      mask Type: Wcdma Rake Combiner
      mask Description: Performs Rake combjner by averaging the output of enabled Rake Fingers blocks.
  Wcdma Rake Finger : Subsystem  TreatAsAtomicUnit=on  EnableExecutionContextPropagation=on  mask(Wcdma Rake Finger){sprdFactor=256, overSampling=8, numChipsOut=256, st=1/15e3}
      mask prompts: sprdFactor "DPCH Spreading Factor (SF):"; overSampling "Oversampling Factor:"; numChipsOut "Number of Chips per Output:"; st "Sampling Time:"
      mask help: Each finger downsamples and decorrelates pilot bits and data using the corresponding channelization code and Gold Code sequence.
      mask init:
      | numSymbOut = numChipsOut/256;
      mask Help: Each finger downsamples and decorrelates pilot bits and data using the corresponding channelization code and Gold Code sequence.
  Wcdma Rake Receiver : Subsystem  EnableExecutionContextPropagation=on  mask(Wcdma Rake Receiver){sprdFactor=256, codeNumber=256-1, scrCode=[63 0], numTapsChEst=3, numTapsRRC=32, overSampling=8, fingerEnables=[1 0 0 0], fingerPhases=[0 0 0 0], numChipsOut=256, st=1/15e3}
      mask prompts: sprdFactor "DPCH Spreading Factor (SF):"; codeNumber "Code Number (k):"; scrCode "Scrambling Code [Scr Code Grup(0..63)  Primary Code(0..7)]:"; numTapsChEst "Number of Filter Taps for Channel Estimation:"; numTapsRRC "Number of Filter Taps for RRC filters:"; overSampling "Oversampling Factor:"; fingerEnables "Finger Enables:"; fingerPhases "Finger Phases (in units of Ticks):"; numChipsOut "Number of Chips per Output:"; st "Symbol Time (Ts):"
      mask help:
      | Rake receiver is made of 4 different fingers. Each finger downsamples and decorrelates pilot bits and data using the corresponding channelization code and Gold Code sequence.
      |
      | Pilot bits are then sent to the channel estimator whose output is then used to derotate the received data signal. The demodulated data processed by each rake finger is finally coherently combined before sending it to the physical channel demapping.
      mask init:
      | numSymbOut = numChipsOut/256;
      | st =  numSymbOut*st;
      | 
      | % Setting Parameters
      | numTapsRRC = numTapsRRC - (mod(numTapsRRC,2));
      | numSymbFrame = numChipsOut/sprdFactor;
      | rxTicksDelay = numTapsRRC + fingerPhases;
      | rxSymDelay = ceil(rxTicksDelay/(numChipsOut*overSampling));
      | maxSymDelay = max(rxSymDelay*diag(fingerEnables));
      mask Help:
      | <p>Rake receiver is made of 4 different fingers. Each finger downsamples and decorrelates pilot bits and data using the corresponding channelization code and Gold Code sequence. </p>
      | 
      | <p>Pilot bits are then sent to the channel estimator whose output is then used to derotate the received data signal. The demodulated data processed by each rake finger is finally coherently combined before sending it to the physical channel demapping.</p>
      mask Display: disp('RAKE Receiver');
  Wcdma UE Rx Antenna : Subsystem  EnableExecutionContextPropagation=on  mask(Wcdma UE Rx Antenna){slotFormat=11, dpchCode=127, scrCode=[63 0], powerVector=[-16.6 -10 -15 -12 -12], numTapsRRC=32, overSampling=8, fingerEnables=[1 0 0 0], fingerPhases=[0 0 0 0], numTapsChEst=31, checkParams=off}
      mask prompts: slotFormat "Slot Format (0..16):"; dpchCode "DPCH Code number (0..Spreading Factor -1):"; scrCode "Scrambling Code [Scr Code Grup(0..63) Primary Code(0..7)]:"; powerVector "Power for [DPCH, P-CPICH, PICH, P-CCPCH, SCH] in dB:"; numTapsRRC "Number of Filter Taps for RRC filters:"; overSampling "Oversampling Factor:"; fingerEnables "Finger Enables:"; fingerPhases "Finger Phases (in s):"; numTapsChEst "Number of Filter Taps for Channel Estimation:"; checkParams "Check here to validate parameters."
      mask help:
      | After applying the receiver pulse shaping filter, oversampled data is sent to the Rake receiver.
      |
      | Rake receiver is made of 4 different fingers. Each finger downsamples and decorrelates pilot bits and data using the corresponding channelization code and Gold Code sequence.
      |
      | Pilot bits are then sent to the channel estimator whose output is then use to derotate the received data signal. The demodulated data processed by each rake finger is finally coherently combined before sending it to the physical channel demapping.
      |
      | For details on the implementation, see 3GPP TS 25.101, 3GPP TS 25.211 and 3GPP TS 25.213.
      mask init:
      | if slotFormat < 2
      | numChipsOut = 512;
      | else
      | numChipsOut = 256;
      | end
      | 
      | load wcdma_slotformattable;
      | sprdFactor = slotformattable(slotFormat+1,2);
      | numSymbOut = numChipsOut/sprdFactor;
      | numBits = slotformattable(slotFormat+1,3);
      | 
      | len = length(fingerPhases);
      | fingerPhases = [fingerPhases zeros(1,4-len)];
      | fingerPhases = round(fingerPhases*3.84e6*overSampling);
      | 
      | % Compute Total Received Delay
      | latestPath = max(fingerPhases);
      | filtDelayChEst = (numTapsChEst-1)/2;
      | rxDelayinFrames = ceil(((numTapsRRC/overSampling)+latestPath)/numChipsOut) + filtDelayChEst;
      | rxDelay = rxDelayinFrames * numSymbOut;
      | rxSlotsDelay = ceil(rxDelay*2/numBits);
      | 
      | % Check parameters
      | if(checkParams == 1)
      | wcdma_checkparamsrxant;
      | end
      mask Help:
      | <p>After applying the receiver pulse shaping filter, oversampled data is sent to the Rake receiver. </p>
      | <p>Rake receiver is made of 4 different fingers. Each finger downsamples and decorrelates pilot bits and data using the corresponding channelization code and Gold Code sequence. </p>
      | <p>Pilot bits are then sent to the channel estimator whose output is then use to derotate the received data signal. The demodulated data processed by each rake finger is finally coherently combined before sending it to the physical channel demapping.</p>
      | <p>For details on the implementation, see <a href="http://www.3gpp.org/specs/download.htm">3GPP TS.101 </a>, <a href="http://www.3gpp.org/specs/download.htm"> 3GPP TS 25.211</a> and <a href="http://www.3gpp.org/specs/download.htm"> 3GPP TS 25.213</a>.</p>
      mask Display: disp('Wcdma UE Rx\nAntenna');

== system wcdma_lib/Wcdma BS Transmitter/Complex Spreading Multiplication ==
  cIn : Inport  LatchInput=off
  Channel Code : Inport  Port=2  LatchInput=off
  Product : Product  SaturateOnIntegerOverflow=on  InputSameDT=on
  Repeat : dspsigops/Repeat  N=sprdFactor  ic=0  mode=Maintain input frame rate
  cOut : Outport
  wires:
  Repeat/1 -> Product/1
  cIn/1 -> Repeat/1
  Product/1 -> cOut/1
  Channel Code/1 -> Product/2
